simulink model "pid_adrc_duibi"  (R2023b)
settings: Solver=VariableStepAuto  StartTime=0.0  StopTime=10.0  RelTol=1e-3
values from neighbouring files (symbols this model uses):
  gama = 0.003    [startup.m]
  ke = 78.4    [startup.m]
  kf = 96.0    (= 96)    [startup.m]
  kii = 1061*R    (= 19755.82)    [startup.m]
  kiv = kpv*100    (= 7015.3125)    [startup.m]
  kp = 150    [startup.m]
  kpi = 1061*L    (= 16265.13)    [startup.m]
  kpv = 100*6*J/(kf)    (= 70.153125)    [startup.m]
  L = 15.33    [startup.m]
  R = 18.62    [startup.m]
  r = 10    [startup.m]
  tao = 0.003    [startup.m]
  U = m2^2*y^2+2*m1*m2*y^2+I1*(m1+m2)    [startup.m]
undefined symbols (not defined in the file or in its folder): sigbuilder_block
libraries: slpidlib x42, simulink x18
(part 1 of 2)
settings Model: Creator=CAE_B7  LastModifiedBy=Keaton
settings SolverCC: AlgebraicLoopSolver=TrustRegion
settings DataIOCC: ReturnWorkspaceOutputs=off
settings DebuggingCC: UnconnectedInputMsg=warning  UnconnectedOutputMsg=warning  UnconnectedLineMsg=warning  ArithmeticOperatorsInVariantConditions=warning
settings ModelReferenceCC: EnableRefExpFcnMdlSchedulingChecks=on
settings SFSimCC: SimUseLocalCustomCode=off  CustomCodeUndefinedFunction=UseInterfaceOnly
settings RTWCC: RTWUseLocalCustomCode=off

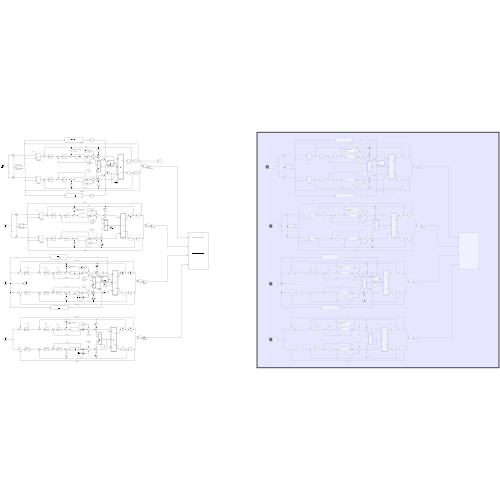
[thumbnail: Simulink's stored preview of the top-level diagram]
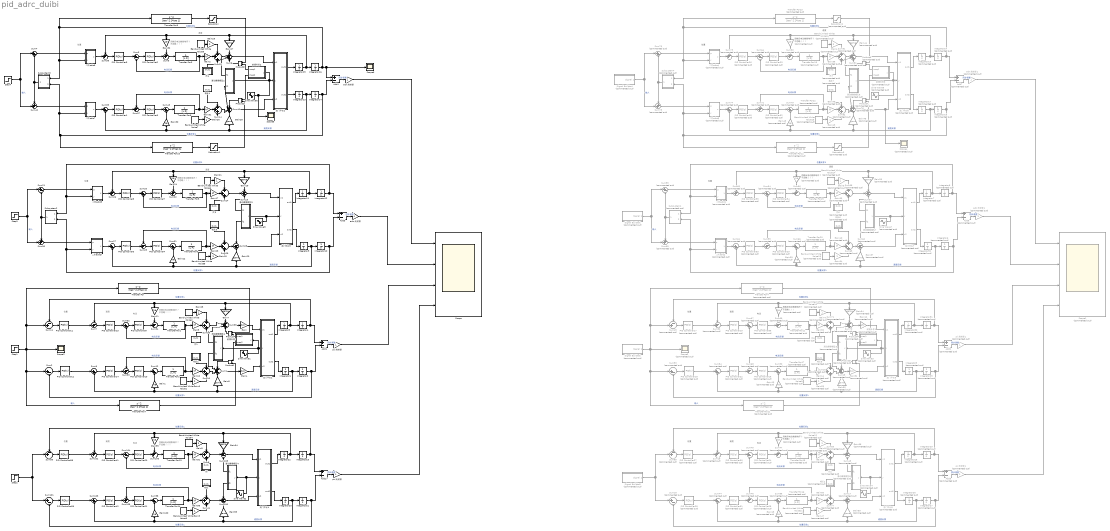
== system pid_adrc_duibi ==
  note: 速度
  note: 位置
  note: 忽略反电动势影响不？
      | 不忽略！！！
  note: 忽略反电动势影响不？
      | 不忽略！！！
  note: 忽略反电动势影响不？
      | 不忽略！！！
  note: 电流
  note: 速度
  note: 位置
  note: 位置
  note: 电流
  note: 速度
  note: 速度
  note: 位置
  note: 忽略反电动势影响不？
      | 不忽略！！！
  note: 忽略反电动势影响不？
      | 不忽略！！！
  note: 位置
  note: 电流
  note: 速度
  note: 位置
  note: 速度
  note: 电流
  note: 速度
  note: 忽略反电动势影响不？
      | 不忽略！！！
  note: 位置
  note: 速度
  note: 忽略反电动势影响不？
      | 不忽略！！！
  note: 位置
  note: 忽略反电动势影响不？
      | 不忽略！！！
  Add{1,3..4,17} (4 alike) : Sum  Inputs=+-
  Add{2,5..7} (4 alike) : Sum  Commented=on  Inputs=+-
  Band-Limited White Noise{1,3,5,7} (4 alike) : simulink/Sources/Band-Limited White Noise  Cov=[0.0001]  Ts=0.0001  seed=[23342]
  Band-Limited White Noise{10,12,14,16} (4 alike) : simulink/Sources/Band-Limited White Noise  Commented=on  Cov=[0.0001]  Ts=0.0001  seed=[23341]
  Band-Limited White Noise{9,11,13,15} (4 alike) : simulink/Sources/Band-Limited White Noise  Commented=on  Cov=[0.0001]  Ts=0.0001  seed=[23342]
  Band-Limited White Noise{2,4,6,8} (4 alike) : simulink/Sources/Band-Limited White Noise  Cov=[0.0001]  Ts=0.0001  seed=[23341]
  Gain : Gain  Gain=1/U
  Gain{1,11,22,24,30,32,99..100} (8 alike) : Gain  Gain=ke
  Gain{2,5,10,17,23,31,92,98} (8 alike) : Gain  Gain=kf
  Gain12 : Gain  Commented=on  Gain=1/U
  Gain{13,15..16,39,41,48,50,61} (8 alike) : Gain  Commented=on  Gain=ke
  Gain{14,33,36,40,49,52,57,60} (8 alike) : Gain  Commented=on  Gain=kf
  Gain{3,6,9,18,21,25..26,29} (8 alike) : Gain
  Gain{7..8,19..20,27..28,94..95} (8 alike) : Gain  Gain=gama
  Gain{34,38,42..43,46..47,53,56} (8 alike) : Gain  Commented=on
  Gain{35,37,44..45,54..55,58..59} (8 alike) : Gain  Commented=on  Gain=gama
  Gain4 : Gain  Gain=1/U
  Gain51 : Gain  Commented=on  Gain=1/U
  Integrator{1..4,9..16,20..23} (16 alike) : Integrator
  Integrator{5..8,17..19,24..32} (16 alike) : Integrator  Commented=on
  PID Controller{1,3,6,8,13..14,41..42} (8 alike) : slpidlib/PID Controller  Controller=PID  Form=Parallel  TimeDomain=Continuous-time  UseExternalTs=off  SampleTime=-1  IntegratorMethod=Forward Euler  FilterMethod=Forward Euler  ControllerParametersSource=internal  P=kpv  I=kiv  UseKiTs=off  D=0  N=100  UseFilter=on  TunerSelectOption=Transfer Function Based (PID Tuner App)  InitialConditionSource=internal  InitialConditionForIntegrator=0  InitialConditionForFilter=0  DifferentiatorICPrevScaledInput=0  ExternalReset=none  TrackingMode=off  Kt=1  LimitOutput=off  SatLimitsSource=internal  UpperSaturationLimit=inf  LowerSaturationLimit=-inf  LinearizeAsGain=on  AntiWindupMode=none  Kb=1  LimitIntegrator=off  UpperIntegratorSaturationLimit=inf  LowerIntegratorSaturationLimit=-inf  POutMin=[]  POutMax=[]  IOutMin=[]  IOutMax=[]  DOutMin=[]  DOutMax=[]  NOutMin=[]  NOutMax=[]  SumOutMin=[]  SumOutMax=[]  SaturationOutMin=[]  SaturationOutMax=[]  PParamMin=[]  PParamMax=[]  IParamMin=[]  IParamMax=[]  DParamMin=[]  DParamMax=[]  NParamMin=[]  NParamMax=[]  KbParamMin=[]  KbParamMax=[]  KtParamMin=[]  KtParamMax=[]  KbOutMin=[]  KbOutMax=[]  KtOutMin=[]  KtOutMax=[]  IntegratorOutMin=[]  IntegratorOutMax=[]  FilterOutMin=[]  FilterOutMax=[]  SumI1OutMin=[]  SumI1OutMax=[]  SumI2OutMin=[]  SumI2OutMax=[]  SumI3OutMin=[]  SumI3OutMax=[]  SumI4OutMin=[]  SumI4OutMax=[]  SumDOutMin=[]  SumDOutMax=[]  DifferentiatorOutMin=[]  DifferentiatorOutMax=[]  FilterDiffOutCoefMin=[]  FilterDiffOutCoefMax=[]  ReciprocalOutMin=[]  ReciprocalOutMax=[]  SumDenOutMin=[]  SumDenOutMax=[]  SumNumOutMin=[]  SumNumOutMax=[]  DivideOutMin=[]  DivideOutMax=[]  UdiffTsProdOutMin=[]  UdiffTsProdOutMax=[]  NTsProdOutMin=[]  NTsProdOutMax=[]  UintegralTsProdOutMin=[]  UintegralTsProdOutMax=[]  UngainTsProdOutMin=[]  UngainTsProdOutMax=[]  ClampingZeroOutDataTypeStr=Inherit: Inherit via back propagation  ClampingZeroOutMin=[]  ClampingZeroOutMax=[]  FilterDenConstantOutDataTypeStr=Inherit: Inherit via back propagation  FilterDenConstantOutMin=[]  FilterDenConstantOutMax=[]  PCopyOutDataTypeStr=Inherit: Inherit via back propagation  PCopyOutMin=[]  PCopyOutMax=[]  NCopyOutDataTypeStr=Inherit: Inherit via back propagation  NCopyOutMin=[]  NCopyOutMax=[]  IntegratorContinuousStateAttributes=''  IntegratorStateMustResolveToSignalObject=off  IntegratorRTWStateStorageClass=Auto  FilterContinuousStateAttributes=''  FilterStateMustResolveToSignalObject=off  FilterRTWStateStorageClass=Auto  ParallelPVariant=InternalParameters  IdealPVariant=Disabled  IVariant=InternalParameters  DVariant=InternalParameters  IntegratorVariant=Continuous  SatVariant=Disabled  AWVariant=Passthrough  PCopyVariant=Disabled  TRVariant=Disabled  FdbkBlocksVariant=Forward  IdealPFdbkVariant=Disabled  SatFdbkVariant=Disabled  DerivativeFilterVariant=ContFilter  NVariant=InternalParameters  NCopyVariant=Disabled  FilterICVariant=InternalICsFilter  IntegratorICVariant=InternalICs  ExternalResetVariant=Disabled  TRSumVariant=Passthrough  SumFdbkVariant=Disabled  SumVariant=Sum_PID  TsampFilterVariant=InternalTs  TsampNgainVariant=Passthrough  TsampIntegralVariant=Disabled_SignalSpec  ExternalSaturationOutDataTypeStr=Inherit: Same as second input
  PID Controller{2,4..5,7,9..10,20..21} (8 alike) : slpidlib/PID Controller  Controller=PID  Form=Parallel  TimeDomain=Continuous-time  UseExternalTs=off  SampleTime=-1  IntegratorMethod=Forward Euler  FilterMethod=Forward Euler  ControllerParametersSource=internal  P=kpi  I=kii  UseKiTs=off  D=0  N=100  UseFilter=on  TunerSelectOption=Transfer Function Based (PID Tuner App)  InitialConditionSource=internal  InitialConditionForIntegrator=0  InitialConditionForFilter=0  DifferentiatorICPrevScaledInput=0  ExternalReset=none  TrackingMode=off  Kt=1  LimitOutput=off  SatLimitsSource=internal  UpperSaturationLimit=inf  LowerSaturationLimit=-inf  LinearizeAsGain=on  AntiWindupMode=none  Kb=1  LimitIntegrator=off  UpperIntegratorSaturationLimit=inf  LowerIntegratorSaturationLimit=-inf  POutMin=[]  POutMax=[]  IOutMin=[]  IOutMax=[]  DOutMin=[]  DOutMax=[]  NOutMin=[]  NOutMax=[]  SumOutMin=[]  SumOutMax=[]  SaturationOutMin=[]  SaturationOutMax=[]  PParamMin=[]  PParamMax=[]  IParamMin=[]  IParamMax=[]  DParamMin=[]  DParamMax=[]  NParamMin=[]  NParamMax=[]  KbParamMin=[]  KbParamMax=[]  KtParamMin=[]  KtParamMax=[]  KbOutMin=[]  KbOutMax=[]  KtOutMin=[]  KtOutMax=[]  IntegratorOutMin=[]  IntegratorOutMax=[]  FilterOutMin=[]  FilterOutMax=[]  SumI1OutMin=[]  SumI1OutMax=[]  SumI2OutMin=[]  SumI2OutMax=[]  SumI3OutMin=[]  SumI3OutMax=[]  SumI4OutMin=[]  SumI4OutMax=[]  SumDOutMin=[]  SumDOutMax=[]  DifferentiatorOutMin=[]  DifferentiatorOutMax=[]  FilterDiffOutCoefMin=[]  FilterDiffOutCoefMax=[]  ReciprocalOutMin=[]  ReciprocalOutMax=[]  SumDenOutMin=[]  SumDenOutMax=[]  SumNumOutMin=[]  SumNumOutMax=[]  DivideOutMin=[]  DivideOutMax=[]  UdiffTsProdOutMin=[]  UdiffTsProdOutMax=[]  NTsProdOutMin=[]  NTsProdOutMax=[]  UintegralTsProdOutMin=[]  UintegralTsProdOutMax=[]  UngainTsProdOutMin=[]  UngainTsProdOutMax=[]  ClampingZeroOutDataTypeStr=Inherit: Inherit via back propagation  ClampingZeroOutMin=[]  ClampingZeroOutMax=[]  FilterDenConstantOutDataTypeStr=Inherit: Inherit via back propagation  FilterDenConstantOutMin=[]  FilterDenConstantOutMax=[]  PCopyOutDataTypeStr=Inherit: Inherit via back propagation  PCopyOutMin=[]  PCopyOutMax=[]  NCopyOutDataTypeStr=Inherit: Inherit via back propagation  NCopyOutMin=[]  NCopyOutMax=[]  IntegratorContinuousStateAttributes=''  IntegratorStateMustResolveToSignalObject=off  IntegratorRTWStateStorageClass=Auto  FilterContinuousStateAttributes=''  FilterStateMustResolveToSignalObject=off  FilterRTWStateStorageClass=Auto  ParallelPVariant=InternalParameters  IdealPVariant=Disabled  IVariant=InternalParameters  DVariant=InternalParameters  IntegratorVariant=Continuous  SatVariant=Disabled  AWVariant=Passthrough  PCopyVariant=Disabled  TRVariant=Disabled  FdbkBlocksVariant=Forward  IdealPFdbkVariant=Disabled  SatFdbkVariant=Disabled  DerivativeFilterVariant=ContFilter  NVariant=InternalParameters  NCopyVariant=Disabled  FilterICVariant=InternalICsFilter  IntegratorICVariant=InternalICs  ExternalResetVariant=Disabled  TRSumVariant=Passthrough  SumFdbkVariant=Disabled  SumVariant=Sum_PID  TsampFilterVariant=InternalTs  TsampNgainVariant=Passthrough  TsampIntegralVariant=Disabled_SignalSpec  ExternalSaturationOutDataTypeStr=Inherit: Same as second input
  PID Controller11 : slpidlib/PID Controller  Controller=PID  Form=Parallel  TimeDomain=Continuous-time  UseExternalTs=off  SampleTime=-1  IntegratorMethod=Forward Euler  FilterMethod=Forward Euler  ControllerParametersSource=internal  P=kp  I=0  UseKiTs=off  D=0  N=100  UseFilter=on  TunerSelectOption=Transfer Function Based (PID Tuner App)  InitialConditionSource=internal  InitialConditionForIntegrator=0  InitialConditionForFilter=0  DifferentiatorICPrevScaledInput=0  ExternalReset=none  TrackingMode=off  Kt=1  LimitOutput=off  SatLimitsSource=internal  UpperSaturationLimit=inf  LowerSaturationLimit=-inf  LinearizeAsGain=on  AntiWindupMode=none  Kb=1  LimitIntegrator=off  UpperIntegratorSaturationLimit=inf  LowerIntegratorSaturationLimit=-inf  POutMin=[]  POutMax=[]  IOutMin=[]  IOutMax=[]  DOutMin=[]  DOutMax=[]  NOutMin=[]  NOutMax=[]  SumOutMin=[]  SumOutMax=[]  SaturationOutMin=[]  SaturationOutMax=[]  PParamMin=[]  PParamMax=[]  IParamMin=[]  IParamMax=[]  DParamMin=[]  DParamMax=[]  NParamMin=[]  NParamMax=[]  KbParamMin=[]  KbParamMax=[]  KtParamMin=[]  KtParamMax=[]  KbOutMin=[]  KbOutMax=[]  KtOutMin=[]  KtOutMax=[]  IntegratorOutMin=[]  IntegratorOutMax=[]  FilterOutMin=[]  FilterOutMax=[]  SumI1OutMin=[]  SumI1OutMax=[]  SumI2OutMin=[]  SumI2OutMax=[]  SumI3OutMin=[]  SumI3OutMax=[]  SumI4OutMin=[]  SumI4OutMax=[]  SumDOutMin=[]  SumDOutMax=[]  DifferentiatorOutMin=[]  DifferentiatorOutMax=[]  FilterDiffOutCoefMin=[]  FilterDiffOutCoefMax=[]  ReciprocalOutMin=[]  ReciprocalOutMax=[]  SumDenOutMin=[]  SumDenOutMax=[]  SumNumOutMin=[]  SumNumOutMax=[]  DivideOutMin=[]  DivideOutMax=[]  UdiffTsProdOutMin=[]  UdiffTsProdOutMax=[]  NTsProdOutMin=[]  NTsProdOutMax=[]  UintegralTsProdOutMin=[]  UintegralTsProdOutMax=[]  UngainTsProdOutMin=[]  UngainTsProdOutMax=[]  ClampingZeroOutDataTypeStr=Inherit: Inherit via back propagation  ClampingZeroOutMin=[]  ClampingZeroOutMax=[]  FilterDenConstantOutDataTypeStr=Inherit: Inherit via back propagation  FilterDenConstantOutMin=[]  FilterDenConstantOutMax=[]  PCopyOutDataTypeStr=Inherit: Inherit via back propagation  PCopyOutMin=[]  PCopyOutMax=[]  NCopyOutDataTypeStr=Inherit: Inherit via back propagation  NCopyOutMin=[]  NCopyOutMax=[]  IntegratorContinuousStateAttributes=''  IntegratorStateMustResolveToSignalObject=off  IntegratorRTWStateStorageClass=Auto  FilterContinuousStateAttributes=''  FilterStateMustResolveToSignalObject=off  FilterRTWStateStorageClass=Auto  ParallelPVariant=InternalParameters  IdealPVariant=Disabled  IVariant=InternalParameters  DVariant=InternalParameters  IntegratorVariant=Continuous  SatVariant=Disabled  AWVariant=Passthrough  PCopyVariant=Disabled  TRVariant=Disabled  FdbkBlocksVariant=Forward  IdealPFdbkVariant=Disabled  SatFdbkVariant=Disabled  DerivativeFilterVariant=ContFilter  NVariant=InternalParameters  NCopyVariant=Disabled  FilterICVariant=InternalICsFilter  IntegratorICVariant=InternalICs  ExternalResetVariant=Disabled  TRSumVariant=Passthrough  SumFdbkVariant=Disabled  SumVariant=Sum_PID  TsampFilterVariant=InternalTs  TsampNgainVariant=Passthrough  TsampIntegralVariant=Disabled_SignalSpec  ExternalSaturationOutDataTypeStr=Inherit: Same as second input
  PID Controller12 : slpidlib/PID Controller  Controller=PID  Form=Parallel  TimeDomain=Continuous-time  UseExternalTs=off  SampleTime=-1  IntegratorMethod=Forward Euler  FilterMethod=Forward Euler  ControllerParametersSource=internal  P=kp  I=0  UseKiTs=off  D=0  N=95.162581964040484  UseFilter=on  TunerSelectOption=Transfer Function Based (PID Tuner App)  InitialConditionSource=internal  InitialConditionForIntegrator=0  InitialConditionForFilter=0  DifferentiatorICPrevScaledInput=0  ExternalReset=none  TrackingMode=off  Kt=1  LimitOutput=off  SatLimitsSource=internal  UpperSaturationLimit=inf  LowerSaturationLimit=-inf  LinearizeAsGain=on  AntiWindupMode=none  Kb=1  LimitIntegrator=off  UpperIntegratorSaturationLimit=inf  LowerIntegratorSaturationLimit=-inf  POutMin=[]  POutMax=[]  IOutMin=[]  IOutMax=[]  DOutMin=[]  DOutMax=[]  NOutMin=[]  NOutMax=[]  SumOutMin=[]  SumOutMax=[]  SaturationOutMin=[]  SaturationOutMax=[]  PParamMin=[]  PParamMax=[]  IParamMin=[]  IParamMax=[]  DParamMin=[]  DParamMax=[]  NParamMin=[]  NParamMax=[]  KbParamMin=[]  KbParamMax=[]  KtParamMin=[]  KtParamMax=[]  KbOutMin=[]  KbOutMax=[]  KtOutMin=[]  KtOutMax=[]  IntegratorOutMin=[]  IntegratorOutMax=[]  FilterOutMin=[]  FilterOutMax=[]  SumI1OutMin=[]  SumI1OutMax=[]  SumI2OutMin=[]  SumI2OutMax=[]  SumI3OutMin=[]  SumI3OutMax=[]  SumI4OutMin=[]  SumI4OutMax=[]  SumDOutMin=[]  SumDOutMax=[]  DifferentiatorOutMin=[]  DifferentiatorOutMax=[]  FilterDiffOutCoefMin=[]  FilterDiffOutCoefMax=[]  ReciprocalOutMin=[]  ReciprocalOutMax=[]  SumDenOutMin=[]  SumDenOutMax=[]  SumNumOutMin=[]  SumNumOutMax=[]  DivideOutMin=[]  DivideOutMax=[]  UdiffTsProdOutMin=[]  UdiffTsProdOutMax=[]  NTsProdOutMin=[]  NTsProdOutMax=[]  UintegralTsProdOutMin=[]  UintegralTsProdOutMax=[]  UngainTsProdOutMin=[]  UngainTsProdOutMax=[]  ClampingZeroOutDataTypeStr=Inherit: Inherit via back propagation  ClampingZeroOutMin=[]  ClampingZeroOutMax=[]  FilterDenConstantOutDataTypeStr=Inherit: Inherit via back propagation  FilterDenConstantOutMin=[]  FilterDenConstantOutMax=[]  PCopyOutDataTypeStr=Inherit: Inherit via back propagation  PCopyOutMin=[]  PCopyOutMax=[]  NCopyOutDataTypeStr=Inherit: Inherit via back propagation  NCopyOutMin=[]  NCopyOutMax=[]  IntegratorContinuousStateAttributes=''  IntegratorStateMustResolveToSignalObject=off  IntegratorRTWStateStorageClass=Auto  FilterContinuousStateAttributes=''  FilterStateMustResolveToSignalObject=off  FilterRTWStateStorageClass=Auto  ParallelPVariant=InternalParameters  IdealPVariant=Disabled  IVariant=InternalParameters  DVariant=InternalParameters  IntegratorVariant=Continuous  SatVariant=Disabled  AWVariant=Passthrough  PCopyVariant=Disabled  TRVariant=Disabled  FdbkBlocksVariant=Forward  IdealPFdbkVariant=Disabled  SatFdbkVariant=Disabled  DerivativeFilterVariant=ContFilter  NVariant=InternalParameters  NCopyVariant=Disabled  FilterICVariant=InternalICsFilter  IntegratorICVariant=InternalICs  ExternalResetVariant=Disabled  TRSumVariant=Passthrough  SumFdbkVariant=Disabled  SumVariant=Sum_PID  TsampFilterVariant=InternalTs  TsampNgainVariant=Passthrough  TsampIntegralVariant=Disabled_SignalSpec  ExternalSaturationOutDataTypeStr=Inherit: Same as second input
  PID Controller{15,19,22,26,30..31,33,35} (8 alike) : slpidlib/PID Controller  Commented=on  Controller=PID  Form=Parallel  TimeDomain=Continuous-time  UseExternalTs=off  SampleTime=-1  IntegratorMethod=Forward Euler  FilterMethod=Forward Euler  ControllerParametersSource=internal  P=kpv  I=kiv  UseKiTs=off  D=0  N=100  UseFilter=on  TunerSelectOption=Transfer Function Based (PID Tuner App)  InitialConditionSource=internal  InitialConditionForIntegrator=0  InitialConditionForFilter=0  DifferentiatorICPrevScaledInput=0  ExternalReset=none  TrackingMode=off  Kt=1  LimitOutput=off  SatLimitsSource=internal  UpperSaturationLimit=inf  LowerSaturationLimit=-inf  LinearizeAsGain=on  AntiWindupMode=none  Kb=1  LimitIntegrator=off  UpperIntegratorSaturationLimit=inf  LowerIntegratorSaturationLimit=-inf  POutMin=[]  POutMax=[]  IOutMin=[]  IOutMax=[]  DOutMin=[]  DOutMax=[]  NOutMin=[]  NOutMax=[]  SumOutMin=[]  SumOutMax=[]  SaturationOutMin=[]  SaturationOutMax=[]  PParamMin=[]  PParamMax=[]  IParamMin=[]  IParamMax=[]  DParamMin=[]  DParamMax=[]  NParamMin=[]  NParamMax=[]  KbParamMin=[]  KbParamMax=[]  KtParamMin=[]  KtParamMax=[]  KbOutMin=[]  KbOutMax=[]  KtOutMin=[]  KtOutMax=[]  IntegratorOutMin=[]  IntegratorOutMax=[]  FilterOutMin=[]  FilterOutMax=[]  SumI1OutMin=[]  SumI1OutMax=[]  SumI2OutMin=[]  SumI2OutMax=[]  SumI3OutMin=[]  SumI3OutMax=[]  SumI4OutMin=[]  SumI4OutMax=[]  SumDOutMin=[]  SumDOutMax=[]  DifferentiatorOutMin=[]  DifferentiatorOutMax=[]  FilterDiffOutCoefMin=[]  FilterDiffOutCoefMax=[]  ReciprocalOutMin=[]  ReciprocalOutMax=[]  SumDenOutMin=[]  SumDenOutMax=[]  SumNumOutMin=[]  SumNumOutMax=[]  DivideOutMin=[]  DivideOutMax=[]  UdiffTsProdOutMin=[]  UdiffTsProdOutMax=[]  NTsProdOutMin=[]  NTsProdOutMax=[]  UintegralTsProdOutMin=[]  UintegralTsProdOutMax=[]  UngainTsProdOutMin=[]  UngainTsProdOutMax=[]  ClampingZeroOutDataTypeStr=Inherit: Inherit via back propagation  ClampingZeroOutMin=[]  ClampingZeroOutMax=[]  FilterDenConstantOutDataTypeStr=Inherit: Inherit via back propagation  FilterDenConstantOutMin=[]  FilterDenConstantOutMax=[]  PCopyOutDataTypeStr=Inherit: Inherit via back propagation  PCopyOutMin=[]  PCopyOutMax=[]  NCopyOutDataTypeStr=Inherit: Inherit via back propagation  NCopyOutMin=[]  NCopyOutMax=[]  IntegratorContinuousStateAttributes=''  IntegratorStateMustResolveToSignalObject=off  IntegratorRTWStateStorageClass=Auto  FilterContinuousStateAttributes=''  FilterStateMustResolveToSignalObject=off  FilterRTWStateStorageClass=Auto  ParallelPVariant=InternalParameters  IdealPVariant=Disabled  IVariant=InternalParameters  DVariant=InternalParameters  IntegratorVariant=Continuous  SatVariant=Disabled  AWVariant=Passthrough  PCopyVariant=Disabled  TRVariant=Disabled  FdbkBlocksVariant=Forward  IdealPFdbkVariant=Disabled  SatFdbkVariant=Disabled  DerivativeFilterVariant=ContFilter  NVariant=InternalParameters  NCopyVariant=Disabled  FilterICVariant=InternalICsFilter  IntegratorICVariant=InternalICs  ExternalResetVariant=Disabled  TRSumVariant=Passthrough  SumFdbkVariant=Disabled  SumVariant=Sum_PID  TsampFilterVariant=InternalTs  TsampNgainVariant=Passthrough  TsampIntegralVariant=Disabled_SignalSpec  ExternalSaturationOutDataTypeStr=Inherit: Same as second input
  PID Controller{16,23..25,29,32,34,36} (8 alike) : slpidlib/PID Controller  Commented=on  Controller=PID  Form=Parallel  TimeDomain=Continuous-time  UseExternalTs=off  SampleTime=-1  IntegratorMethod=Forward Euler  FilterMethod=Forward Euler  ControllerParametersSource=internal  P=kpi  I=kii  UseKiTs=off  D=0  N=100  UseFilter=on  TunerSelectOption=Transfer Function Based (PID Tuner App)  InitialConditionSource=internal  InitialConditionForIntegrator=0  InitialConditionForFilter=0  DifferentiatorICPrevScaledInput=0  ExternalReset=none  TrackingMode=off  Kt=1  LimitOutput=off  SatLimitsSource=internal  UpperSaturationLimit=inf  LowerSaturationLimit=-inf  LinearizeAsGain=on  AntiWindupMode=none  Kb=1  LimitIntegrator=off  UpperIntegratorSaturationLimit=inf  LowerIntegratorSaturationLimit=-inf  POutMin=[]  POutMax=[]  IOutMin=[]  IOutMax=[]  DOutMin=[]  DOutMax=[]  NOutMin=[]  NOutMax=[]  SumOutMin=[]  SumOutMax=[]  SaturationOutMin=[]  SaturationOutMax=[]  PParamMin=[]  PParamMax=[]  IParamMin=[]  IParamMax=[]  DParamMin=[]  DParamMax=[]  NParamMin=[]  NParamMax=[]  KbParamMin=[]  KbParamMax=[]  KtParamMin=[]  KtParamMax=[]  KbOutMin=[]  KbOutMax=[]  KtOutMin=[]  KtOutMax=[]  IntegratorOutMin=[]  IntegratorOutMax=[]  FilterOutMin=[]  FilterOutMax=[]  SumI1OutMin=[]  SumI1OutMax=[]  SumI2OutMin=[]  SumI2OutMax=[]  SumI3OutMin=[]  SumI3OutMax=[]  SumI4OutMin=[]  SumI4OutMax=[]  SumDOutMin=[]  SumDOutMax=[]  DifferentiatorOutMin=[]  DifferentiatorOutMax=[]  FilterDiffOutCoefMin=[]  FilterDiffOutCoefMax=[]  ReciprocalOutMin=[]  ReciprocalOutMax=[]  SumDenOutMin=[]  SumDenOutMax=[]  SumNumOutMin=[]  SumNumOutMax=[]  DivideOutMin=[]  DivideOutMax=[]  UdiffTsProdOutMin=[]  UdiffTsProdOutMax=[]  NTsProdOutMin=[]  NTsProdOutMax=[]  UintegralTsProdOutMin=[]  UintegralTsProdOutMax=[]  UngainTsProdOutMin=[]  UngainTsProdOutMax=[]  ClampingZeroOutDataTypeStr=Inherit: Inherit via back propagation  ClampingZeroOutMin=[]  ClampingZeroOutMax=[]  FilterDenConstantOutDataTypeStr=Inherit: Inherit via back propagation  FilterDenConstantOutMin=[]  FilterDenConstantOutMax=[]  PCopyOutDataTypeStr=Inherit: Inherit via back propagation  PCopyOutMin=[]  PCopyOutMax=[]  NCopyOutDataTypeStr=Inherit: Inherit via back propagation  NCopyOutMin=[]  NCopyOutMax=[]  IntegratorContinuousStateAttributes=''  IntegratorStateMustResolveToSignalObject=off  IntegratorRTWStateStorageClass=Auto  FilterContinuousStateAttributes=''  FilterStateMustResolveToSignalObject=off  FilterRTWStateStorageClass=Auto  ParallelPVariant=InternalParameters  IdealPVariant=Disabled  IVariant=InternalParameters  DVariant=InternalParameters  IntegratorVariant=Continuous  SatVariant=Disabled  AWVariant=Passthrough  PCopyVariant=Disabled  TRVariant=Disabled  FdbkBlocksVariant=Forward  IdealPFdbkVariant=Disabled  SatFdbkVariant=Disabled  DerivativeFilterVariant=ContFilter  NVariant=InternalParameters  NCopyVariant=Disabled  FilterICVariant=InternalICsFilter  IntegratorICVariant=InternalICs  ExternalResetVariant=Disabled  TRSumVariant=Passthrough  SumFdbkVariant=Disabled  SumVariant=Sum_PID  TsampFilterVariant=InternalTs  TsampNgainVariant=Passthrough  TsampIntegralVariant=Disabled_SignalSpec  ExternalSaturationOutDataTypeStr=Inherit: Same as second input
  PID Controller17 : slpidlib/PID Controller  Commented=on  Controller=PID  Form=Parallel  TimeDomain=Continuous-time  UseExternalTs=off  SampleTime=-1  IntegratorMethod=Forward Euler  FilterMethod=Forward Euler  ControllerParametersSource=internal  P=kp  I=0  UseKiTs=off  D=0  N=100  UseFilter=on  TunerSelectOption=Transfer Function Based (PID Tuner App)  InitialConditionSource=internal  InitialConditionForIntegrator=0  InitialConditionForFilter=0  DifferentiatorICPrevScaledInput=0  ExternalReset=none  TrackingMode=off  Kt=1  LimitOutput=off  SatLimitsSource=internal  UpperSaturationLimit=inf  LowerSaturationLimit=-inf  LinearizeAsGain=on  AntiWindupMode=none  Kb=1  LimitIntegrator=off  UpperIntegratorSaturationLimit=inf  LowerIntegratorSaturationLimit=-inf  POutMin=[]  POutMax=[]  IOutMin=[]  IOutMax=[]  DOutMin=[]  DOutMax=[]  NOutMin=[]  NOutMax=[]  SumOutMin=[]  SumOutMax=[]  SaturationOutMin=[]  SaturationOutMax=[]  PParamMin=[]  PParamMax=[]  IParamMin=[]  IParamMax=[]  DParamMin=[]  DParamMax=[]  NParamMin=[]  NParamMax=[]  KbParamMin=[]  KbParamMax=[]  KtParamMin=[]  KtParamMax=[]  KbOutMin=[]  KbOutMax=[]  KtOutMin=[]  KtOutMax=[]  IntegratorOutMin=[]  IntegratorOutMax=[]  FilterOutMin=[]  FilterOutMax=[]  SumI1OutMin=[]  SumI1OutMax=[]  SumI2OutMin=[]  SumI2OutMax=[]  SumI3OutMin=[]  SumI3OutMax=[]  SumI4OutMin=[]  SumI4OutMax=[]  SumDOutMin=[]  SumDOutMax=[]  DifferentiatorOutMin=[]  DifferentiatorOutMax=[]  FilterDiffOutCoefMin=[]  FilterDiffOutCoefMax=[]  ReciprocalOutMin=[]  ReciprocalOutMax=[]  SumDenOutMin=[]  SumDenOutMax=[]  SumNumOutMin=[]  SumNumOutMax=[]  DivideOutMin=[]  DivideOutMax=[]  UdiffTsProdOutMin=[]  UdiffTsProdOutMax=[]  NTsProdOutMin=[]  NTsProdOutMax=[]  UintegralTsProdOutMin=[]  UintegralTsProdOutMax=[]  UngainTsProdOutMin=[]  UngainTsProdOutMax=[]  ClampingZeroOutDataTypeStr=Inherit: Inherit via back propagation  ClampingZeroOutMin=[]  ClampingZeroOutMax=[]  FilterDenConstantOutDataTypeStr=Inherit: Inherit via back propagation  FilterDenConstantOutMin=[]  FilterDenConstantOutMax=[]  PCopyOutDataTypeStr=Inherit: Inherit via back propagation  PCopyOutMin=[]  PCopyOutMax=[]  NCopyOutDataTypeStr=Inherit: Inherit via back propagation  NCopyOutMin=[]  NCopyOutMax=[]  IntegratorContinuousStateAttributes=''  IntegratorStateMustResolveToSignalObject=off  IntegratorRTWStateStorageClass=Auto  FilterContinuousStateAttributes=''  FilterStateMustResolveToSignalObject=off  FilterRTWStateStorageClass=Auto  ParallelPVariant=InternalParameters  IdealPVariant=Disabled  IVariant=InternalParameters  DVariant=InternalParameters  IntegratorVariant=Continuous  SatVariant=Disabled  AWVariant=Passthrough  PCopyVariant=Disabled  TRVariant=Disabled  FdbkBlocksVariant=Forward  IdealPFdbkVariant=Disabled  SatFdbkVariant=Disabled  DerivativeFilterVariant=ContFilter  NVariant=InternalParameters  NCopyVariant=Disabled  FilterICVariant=InternalICsFilter  IntegratorICVariant=InternalICs  ExternalResetVariant=Disabled  TRSumVariant=Passthrough  SumFdbkVariant=Disabled  SumVariant=Sum_PID  TsampFilterVariant=InternalTs  TsampNgainVariant=Passthrough  TsampIntegralVariant=Disabled_SignalSpec  ExternalSaturationOutDataTypeStr=Inherit: Same as second input
  PID Controller18 : slpidlib/PID Controller  Commented=on  Controller=PID  Form=Parallel  TimeDomain=Continuous-time  UseExternalTs=off  SampleTime=-1  IntegratorMethod=Forward Euler  FilterMethod=Forward Euler  ControllerParametersSource=internal  P=kp  I=0  UseKiTs=off  D=0  N=95.162581964040484  UseFilter=on  TunerSelectOption=Transfer Function Based (PID Tuner App)  InitialConditionSource=internal  InitialConditionForIntegrator=0  InitialConditionForFilter=0  DifferentiatorICPrevScaledInput=0  ExternalReset=none  TrackingMode=off  Kt=1  LimitOutput=off  SatLimitsSource=internal  UpperSaturationLimit=inf  LowerSaturationLimit=-inf  LinearizeAsGain=on  AntiWindupMode=none  Kb=1  LimitIntegrator=off  UpperIntegratorSaturationLimit=inf  LowerIntegratorSaturationLimit=-inf  POutMin=[]  POutMax=[]  IOutMin=[]  IOutMax=[]  DOutMin=[]  DOutMax=[]  NOutMin=[]  NOutMax=[]  SumOutMin=[]  SumOutMax=[]  SaturationOutMin=[]  SaturationOutMax=[]  PParamMin=[]  PParamMax=[]  IParamMin=[]  IParamMax=[]  DParamMin=[]  DParamMax=[]  NParamMin=[]  NParamMax=[]  KbParamMin=[]  KbParamMax=[]  KtParamMin=[]  KtParamMax=[]  KbOutMin=[]  KbOutMax=[]  KtOutMin=[]  KtOutMax=[]  IntegratorOutMin=[]  IntegratorOutMax=[]  FilterOutMin=[]  FilterOutMax=[]  SumI1OutMin=[]  SumI1OutMax=[]  SumI2OutMin=[]  SumI2OutMax=[]  SumI3OutMin=[]  SumI3OutMax=[]  SumI4OutMin=[]  SumI4OutMax=[]  SumDOutMin=[]  SumDOutMax=[]  DifferentiatorOutMin=[]  DifferentiatorOutMax=[]  FilterDiffOutCoefMin=[]  FilterDiffOutCoefMax=[]  ReciprocalOutMin=[]  ReciprocalOutMax=[]  SumDenOutMin=[]  SumDenOutMax=[]  SumNumOutMin=[]  SumNumOutMax=[]  DivideOutMin=[]  DivideOutMax=[]  UdiffTsProdOutMin=[]  UdiffTsProdOutMax=[]  NTsProdOutMin=[]  NTsProdOutMax=[]  UintegralTsProdOutMin=[]  UintegralTsProdOutMax=[]  UngainTsProdOutMin=[]  UngainTsProdOutMax=[]  ClampingZeroOutDataTypeStr=Inherit: Inherit via back propagation  ClampingZeroOutMin=[]  ClampingZeroOutMax=[]  FilterDenConstantOutDataTypeStr=Inherit: Inherit via back propagation  FilterDenConstantOutMin=[]  FilterDenConstantOutMax=[]  PCopyOutDataTypeStr=Inherit: Inherit via back propagation  PCopyOutMin=[]  PCopyOutMax=[]  NCopyOutDataTypeStr=Inherit: Inherit via back propagation  NCopyOutMin=[]  NCopyOutMax=[]  IntegratorContinuousStateAttributes=''  IntegratorStateMustResolveToSignalObject=off  IntegratorRTWStateStorageClass=Auto  FilterContinuousStateAttributes=''  FilterStateMustResolveToSignalObject=off  FilterRTWStateStorageClass=Auto  ParallelPVariant=InternalParameters  IdealPVariant=Disabled  IVariant=InternalParameters  DVariant=InternalParameters  IntegratorVariant=Continuous  SatVariant=Disabled  AWVariant=Passthrough  PCopyVariant=Disabled  TRVariant=Disabled  FdbkBlocksVariant=Forward  IdealPFdbkVariant=Disabled  SatFdbkVariant=Disabled  DerivativeFilterVariant=ContFilter  NVariant=InternalParameters  NCopyVariant=Disabled  FilterICVariant=InternalICsFilter  IntegratorICVariant=InternalICs  ExternalResetVariant=Disabled  TRSumVariant=Passthrough  SumFdbkVariant=Disabled  SumVariant=Sum_PID  TsampFilterVariant=InternalTs  TsampNgainVariant=Passthrough  TsampIntegralVariant=Disabled_SignalSpec  ExternalSaturationOutDataTypeStr=Inherit: Same as second input
  PID Controller27 : slpidlib/PID Controller  Commented=on  Controller=PID  Form=Parallel  TimeDomain=Continuous-time  UseExternalTs=off  SampleTime=-1  IntegratorMethod=Forward Euler  FilterMethod=Forward Euler  ControllerParametersSource=internal  P=kp  I=0  UseKiTs=off  D=0  N=100  UseFilter=on  TunerSelectOption=Transfer Function Based (PID Tuner App)  InitialConditionSource=internal  InitialConditionForIntegrator=0  InitialConditionForFilter=0  DifferentiatorICPrevScaledInput=0  ExternalReset=none  TrackingMode=off  Kt=1  LimitOutput=off  SatLimitsSource=internal  UpperSaturationLimit=inf  LowerSaturationLimit=-inf  LinearizeAsGain=on  AntiWindupMode=none  Kb=1  LimitIntegrator=off  UpperIntegratorSaturationLimit=inf  LowerIntegratorSaturationLimit=-inf  POutMin=[]  POutMax=[]  IOutMin=[]  IOutMax=[]  DOutMin=[]  DOutMax=[]  NOutMin=[]  NOutMax=[]  SumOutMin=[]  SumOutMax=[]  SaturationOutMin=[]  SaturationOutMax=[]  PParamMin=[]  PParamMax=[]  IParamMin=[]  IParamMax=[]  DParamMin=[]  DParamMax=[]  NParamMin=[]  NParamMax=[]  KbParamMin=[]  KbParamMax=[]  KtParamMin=[]  KtParamMax=[]  KbOutMin=[]  KbOutMax=[]  KtOutMin=[]  KtOutMax=[]  IntegratorOutMin=[]  IntegratorOutMax=[]  FilterOutMin=[]  FilterOutMax=[]  SumI1OutMin=[]  SumI1OutMax=[]  SumI2OutMin=[]  SumI2OutMax=[]  SumI3OutMin=[]  SumI3OutMax=[]  SumI4OutMin=[]  SumI4OutMax=[]  SumDOutMin=[]  SumDOutMax=[]  DifferentiatorOutMin=[]  DifferentiatorOutMax=[]  FilterDiffOutCoefMin=[]  FilterDiffOutCoefMax=[]  ReciprocalOutMin=[]  ReciprocalOutMax=[]  SumDenOutMin=[]  SumDenOutMax=[]  SumNumOutMin=[]  SumNumOutMax=[]  DivideOutMin=[]  DivideOutMax=[]  UdiffTsProdOutMin=[]  UdiffTsProdOutMax=[]  NTsProdOutMin=[]  NTsProdOutMax=[]  UintegralTsProdOutMin=[]  UintegralTsProdOutMax=[]  UngainTsProdOutMin=[]  UngainTsProdOutMax=[]  ClampingZeroOutDataTypeStr=Inherit: Inherit via back propagation  ClampingZeroOutMin=[]  ClampingZeroOutMax=[]  FilterDenConstantOutDataTypeStr=Inherit: Inherit via back propagation  FilterDenConstantOutMin=[]  FilterDenConstantOutMax=[]  PCopyOutDataTypeStr=Inherit: Inherit via back propagation  PCopyOutMin=[]  PCopyOutMax=[]  NCopyOutDataTypeStr=Inherit: Inherit via back propagation  NCopyOutMin=[]  NCopyOutMax=[]  IntegratorContinuousStateAttributes=''  IntegratorStateMustResolveToSignalObject=off  IntegratorRTWStateStorageClass=Auto  FilterContinuousStateAttributes=''  FilterStateMustResolveToSignalObject=off  FilterRTWStateStorageClass=Auto  ParallelPVariant=InternalParameters  IdealPVariant=Disabled  IVariant=InternalParameters  DVariant=InternalParameters  IntegratorVariant=Continuous  SatVariant=Disabled  AWVariant=Passthrough  PCopyVariant=Disabled  TRVariant=Disabled  FdbkBlocksVariant=Forward  IdealPFdbkVariant=Disabled  SatFdbkVariant=Disabled  DerivativeFilterVariant=ContFilter  NVariant=InternalParameters  NCopyVariant=Disabled  FilterICVariant=InternalICsFilter  IntegratorICVariant=InternalICs  ExternalResetVariant=Disabled  TRSumVariant=Passthrough  SumFdbkVariant=Disabled  SumVariant=Sum_PID  TsampFilterVariant=InternalTs  TsampNgainVariant=Passthrough  TsampIntegralVariant=Disabled_SignalSpec  ExternalSaturationOutDataTypeStr=Inherit: Same as second input
  PID Controller28 : slpidlib/PID Controller  Commented=on  Controller=PID  Form=Parallel  TimeDomain=Continuous-time  UseExternalTs=off  SampleTime=-1  IntegratorMethod=Forward Euler  FilterMethod=Forward Euler  ControllerParametersSource=internal  P=kp  I=0  UseKiTs=off  D=0  N=95.162581964040484  UseFilter=on  TunerSelectOption=Transfer Function Based (PID Tuner App)  InitialConditionSource=internal  InitialConditionForIntegrator=0  InitialConditionForFilter=0  DifferentiatorICPrevScaledInput=0  ExternalReset=none  TrackingMode=off  Kt=1  LimitOutput=off  SatLimitsSource=internal  UpperSaturationLimit=inf  LowerSaturationLimit=-inf  LinearizeAsGain=on  AntiWindupMode=none  Kb=1  LimitIntegrator=off  UpperIntegratorSaturationLimit=inf  LowerIntegratorSaturationLimit=-inf  POutMin=[]  POutMax=[]  IOutMin=[]  IOutMax=[]  DOutMin=[]  DOutMax=[]  NOutMin=[]  NOutMax=[]  SumOutMin=[]  SumOutMax=[]  SaturationOutMin=[]  SaturationOutMax=[]  PParamMin=[]  PParamMax=[]  IParamMin=[]  IParamMax=[]  DParamMin=[]  DParamMax=[]  NParamMin=[]  NParamMax=[]  KbParamMin=[]  KbParamMax=[]  KtParamMin=[]  KtParamMax=[]  KbOutMin=[]  KbOutMax=[]  KtOutMin=[]  KtOutMax=[]  IntegratorOutMin=[]  IntegratorOutMax=[]  FilterOutMin=[]  FilterOutMax=[]  SumI1OutMin=[]  SumI1OutMax=[]  SumI2OutMin=[]  SumI2OutMax=[]  SumI3OutMin=[]  SumI3OutMax=[]  SumI4OutMin=[]  SumI4OutMax=[]  SumDOutMin=[]  SumDOutMax=[]  DifferentiatorOutMin=[]  DifferentiatorOutMax=[]  FilterDiffOutCoefMin=[]  FilterDiffOutCoefMax=[]  ReciprocalOutMin=[]  ReciprocalOutMax=[]  SumDenOutMin=[]  SumDenOutMax=[]  SumNumOutMin=[]  SumNumOutMax=[]  DivideOutMin=[]  DivideOutMax=[]  UdiffTsProdOutMin=[]  UdiffTsProdOutMax=[]  NTsProdOutMin=[]  NTsProdOutMax=[]  UintegralTsProdOutMin=[]  UintegralTsProdOutMax=[]  UngainTsProdOutMin=[]  UngainTsProdOutMax=[]  ClampingZeroOutDataTypeStr=Inherit: Inherit via back propagation  ClampingZeroOutMin=[]  ClampingZeroOutMax=[]  FilterDenConstantOutDataTypeStr=Inherit: Inherit via back propagation  FilterDenConstantOutMin=[]  FilterDenConstantOutMax=[]  PCopyOutDataTypeStr=Inherit: Inherit via back propagation  PCopyOutMin=[]  PCopyOutMax=[]  NCopyOutDataTypeStr=Inherit: Inherit via back propagation  NCopyOutMin=[]  NCopyOutMax=[]  IntegratorContinuousStateAttributes=''  IntegratorStateMustResolveToSignalObject=off  IntegratorRTWStateStorageClass=Auto  FilterContinuousStateAttributes=''  FilterStateMustResolveToSignalObject=off  FilterRTWStateStorageClass=Auto  ParallelPVariant=InternalParameters  IdealPVariant=Disabled  IVariant=InternalParameters  DVariant=InternalParameters  IntegratorVariant=Continuous  SatVariant=Disabled  AWVariant=Passthrough  PCopyVariant=Disabled  TRVariant=Disabled  FdbkBlocksVariant=Forward  IdealPFdbkVariant=Disabled  SatFdbkVariant=Disabled  DerivativeFilterVariant=ContFilter  NVariant=InternalParameters  NCopyVariant=Disabled  FilterICVariant=InternalICsFilter  IntegratorICVariant=InternalICs  ExternalResetVariant=Disabled  TRSumVariant=Passthrough  SumFdbkVariant=Disabled  SumVariant=Sum_PID  TsampFilterVariant=InternalTs  TsampNgainVariant=Passthrough  TsampIntegralVariant=Disabled_SignalSpec  ExternalSaturationOutDataTypeStr=Inherit: Same as second input
  PID Controller38 : slpidlib/PID Controller  Controller=PID  Form=Parallel  TimeDomain=Continuous-time  UseExternalTs=off  SampleTime=-1  IntegratorMethod=Forward Euler  FilterMethod=Forward Euler  ControllerParametersSource=internal  P=kp  I=0  UseKiTs=off  D=0  N=100  UseFilter=on  TunerSelectOption=Transfer Function Based (PID Tuner App)  InitialConditionSource=internal  InitialConditionForIntegrator=0  InitialConditionForFilter=0  DifferentiatorICPrevScaledInput=0  ExternalReset=none  TrackingMode=off  Kt=1  LimitOutput=off  SatLimitsSource=internal  UpperSaturationLimit=inf  LowerSaturationLimit=-inf  LinearizeAsGain=on  AntiWindupMode=none  Kb=1  LimitIntegrator=off  UpperIntegratorSaturationLimit=inf  LowerIntegratorSaturationLimit=-inf  POutMin=[]  POutMax=[]  IOutMin=[]  IOutMax=[]  DOutMin=[]  DOutMax=[]  NOutMin=[]  NOutMax=[]  SumOutMin=[]  SumOutMax=[]  SaturationOutMin=[]  SaturationOutMax=[]  PParamMin=[]  PParamMax=[]  IParamMin=[]  IParamMax=[]  DParamMin=[]  DParamMax=[]  NParamMin=[]  NParamMax=[]  KbParamMin=[]  KbParamMax=[]  KtParamMin=[]  KtParamMax=[]  KbOutMin=[]  KbOutMax=[]  KtOutMin=[]  KtOutMax=[]  IntegratorOutMin=[]  IntegratorOutMax=[]  FilterOutMin=[]  FilterOutMax=[]  SumI1OutMin=[]  SumI1OutMax=[]  SumI2OutMin=[]  SumI2OutMax=[]  SumI3OutMin=[]  SumI3OutMax=[]  SumI4OutMin=[]  SumI4OutMax=[]  SumDOutMin=[]  SumDOutMax=[]  DifferentiatorOutMin=[]  DifferentiatorOutMax=[]  FilterDiffOutCoefMin=[]  FilterDiffOutCoefMax=[]  ReciprocalOutMin=[]  ReciprocalOutMax=[]  SumDenOutMin=[]  SumDenOutMax=[]  SumNumOutMin=[]  SumNumOutMax=[]  DivideOutMin=[]  DivideOutMax=[]  UdiffTsProdOutMin=[]  UdiffTsProdOutMax=[]  NTsProdOutMin=[]  NTsProdOutMax=[]  UintegralTsProdOutMin=[]  UintegralTsProdOutMax=[]  UngainTsProdOutMin=[]  UngainTsProdOutMax=[]  ClampingZeroOutDataTypeStr=Inherit: Inherit via back propagation  ClampingZeroOutMin=[]  ClampingZeroOutMax=[]  FilterDenConstantOutDataTypeStr=Inherit: Inherit via back propagation  FilterDenConstantOutMin=[]  FilterDenConstantOutMax=[]  PCopyOutDataTypeStr=Inherit: Inherit via back propagation  PCopyOutMin=[]  PCopyOutMax=[]  NCopyOutDataTypeStr=Inherit: Inherit via back propagation  NCopyOutMin=[]  NCopyOutMax=[]  IntegratorContinuousStateAttributes=''  IntegratorStateMustResolveToSignalObject=off  IntegratorRTWStateStorageClass=Auto  FilterContinuousStateAttributes=''  FilterStateMustResolveToSignalObject=off  FilterRTWStateStorageClass=Auto  ParallelPVariant=InternalParameters  IdealPVariant=Disabled  IVariant=InternalParameters  DVariant=InternalParameters  IntegratorVariant=Continuous  SatVariant=Disabled  AWVariant=Passthrough  PCopyVariant=Disabled  TRVariant=Disabled  FdbkBlocksVariant=Forward  IdealPFdbkVariant=Disabled  SatFdbkVariant=Disabled  DerivativeFilterVariant=ContFilter  NVariant=InternalParameters  NCopyVariant=Disabled  FilterICVariant=InternalICsFilter  IntegratorICVariant=InternalICs  ExternalResetVariant=Disabled  TRSumVariant=Passthrough  SumFdbkVariant=Disabled  SumVariant=Sum_PID  TsampFilterVariant=InternalTs  TsampNgainVariant=Passthrough  TsampIntegralVariant=Disabled_SignalSpec  ExternalSaturationOutDataTypeStr=Inherit: Same as second input
  PID Controller39 : slpidlib/PID Controller  Controller=PID  Form=Parallel  TimeDomain=Continuous-time  UseExternalTs=off  SampleTime=-1  IntegratorMethod=Forward Euler  FilterMethod=Forward Euler  ControllerParametersSource=internal  P=kp  I=0  UseKiTs=off  D=0  N=95.162581964040484  UseFilter=on  TunerSelectOption=Transfer Function Based (PID Tuner App)  InitialConditionSource=internal  InitialConditionForIntegrator=0  InitialConditionForFilter=0  DifferentiatorICPrevScaledInput=0  ExternalReset=none  TrackingMode=off  Kt=1  LimitOutput=off  SatLimitsSource=internal  UpperSaturationLimit=inf  LowerSaturationLimit=-inf  LinearizeAsGain=on  AntiWindupMode=none  Kb=1  LimitIntegrator=off  UpperIntegratorSaturationLimit=inf  LowerIntegratorSaturationLimit=-inf  POutMin=[]  POutMax=[]  IOutMin=[]  IOutMax=[]  DOutMin=[]  DOutMax=[]  NOutMin=[]  NOutMax=[]  SumOutMin=[]  SumOutMax=[]  SaturationOutMin=[]  SaturationOutMax=[]  PParamMin=[]  PParamMax=[]  IParamMin=[]  IParamMax=[]  DParamMin=[]  DParamMax=[]  NParamMin=[]  NParamMax=[]  KbParamMin=[]  KbParamMax=[]  KtParamMin=[]  KtParamMax=[]  KbOutMin=[]  KbOutMax=[]  KtOutMin=[]  KtOutMax=[]  IntegratorOutMin=[]  IntegratorOutMax=[]  FilterOutMin=[]  FilterOutMax=[]  SumI1OutMin=[]  SumI1OutMax=[]  SumI2OutMin=[]  SumI2OutMax=[]  SumI3OutMin=[]  SumI3OutMax=[]  SumI4OutMin=[]  SumI4OutMax=[]  SumDOutMin=[]  SumDOutMax=[]  DifferentiatorOutMin=[]  DifferentiatorOutMax=[]  FilterDiffOutCoefMin=[]  FilterDiffOutCoefMax=[]  ReciprocalOutMin=[]  ReciprocalOutMax=[]  SumDenOutMin=[]  SumDenOutMax=[]  SumNumOutMin=[]  SumNumOutMax=[]  DivideOutMin=[]  DivideOutMax=[]  UdiffTsProdOutMin=[]  UdiffTsProdOutMax=[]  NTsProdOutMin=[]  NTsProdOutMax=[]  UintegralTsProdOutMin=[]  UintegralTsProdOutMax=[]  UngainTsProdOutMin=[]  UngainTsProdOutMax=[]  ClampingZeroOutDataTypeStr=Inherit: Inherit via back propagation  ClampingZeroOutMin=[]  ClampingZeroOutMax=[]  FilterDenConstantOutDataTypeStr=Inherit: Inherit via back propagation  FilterDenConstantOutMin=[]  FilterDenConstantOutMax=[]  PCopyOutDataTypeStr=Inherit: Inherit via back propagation  PCopyOutMin=[]  PCopyOutMax=[]  NCopyOutDataTypeStr=Inherit: Inherit via back propagation  NCopyOutMin=[]  NCopyOutMax=[]  IntegratorContinuousStateAttributes=''  IntegratorStateMustResolveToSignalObject=off  IntegratorRTWStateStorageClass=Auto  FilterContinuousStateAttributes=''  FilterStateMustResolveToSignalObject=off  FilterRTWStateStorageClass=Auto  ParallelPVariant=InternalParameters  IdealPVariant=Disabled  IVariant=InternalParameters  DVariant=InternalParameters  IntegratorVariant=Continuous  SatVariant=Disabled  AWVariant=Passthrough  PCopyVariant=Disabled  TRVariant=Disabled  FdbkBlocksVariant=Forward  IdealPFdbkVariant=Disabled  SatFdbkVariant=Disabled  DerivativeFilterVariant=ContFilter  NVariant=InternalParameters  NCopyVariant=Disabled  FilterICVariant=InternalICsFilter  IntegratorICVariant=InternalICs  ExternalResetVariant=Disabled  TRSumVariant=Passthrough  SumFdbkVariant=Disabled  SumVariant=Sum_PID  TsampFilterVariant=InternalTs  TsampNgainVariant=Passthrough  TsampIntegralVariant=Disabled_SignalSpec  ExternalSaturationOutDataTypeStr=Inherit: Same as second input
  Product{,1..3} (4 alike) : Product
  Product{4..7} (4 alike) : Product  Commented=on
  Saturation : Saturate  UpperLimit=50  LowerLimit=-50
  Saturation1 : Saturate  UpperLimit=50  LowerLimit=-50
  Saturation2 : Saturate  Commented=on  UpperLimit=50  LowerLimit=-50
  Saturation3 : Saturate  Commented=on  UpperLimit=50  LowerLimit=-50
  Scope : Scope  NumInputPorts=4
  Scope1 : Scope  Commented=on  NumInputPorts=4
  Scope2 : Scope
  Scope3 : Scope  Commented=on
  Scope4 : Scope  Commented=on
  Scope5 : Scope
  Scope6 : Scope
  Signal Builder1 : Subsystem  Tag=STV Subsys  Commented=on  LoadFcn=sigbuilder_block('load');  StartFcn=sigbuilder_block('start');  StopFcn=sigbuilder_block('stop');  ClipboardFcn=sigbuilder_block('clipboard');  mask(Sigbuilder block){tuvar=[0:10]}
      mask help: Simulink:masks:SigbuilderBlock_MD
      mask init:
      | if ~strcmp(get_param(bdroot(gcbh),'SimulationStatus'),'stopped') tuvar = sigbuilder_block('maskInit'); end
      settings: CopyFcn=sigbuilder_block('copy');  DeleteFcn=sigbuilder_block('delete');  ModelCloseFcn=sigbuilder_block('modelClose');  PreSaveFcn=sigbuilder_block('preSave');  PauseFcn=sigbuilder_block('pause');  ContinueFcn=sigbuilder_block('continue');  NameChangeFcn=sigbuilder_block('namechange');  OpenFcn=sigbuilder_block('open',[437.6 199.2 550.4 400 ]);  CloseFcn=sigbuilder_block('close');
      mask Display: plot(0, 0, 100, 100,[2, 2, 32, 32, 2], [68, 8, 8, 68, 68],[32, 2], [38, 38], [32, 19, 2],[53, 60, 44], [32, 17, 17, 2],[16, 16, 31, 31]);txt = getActiveGroup(gcbh);text(2, 100, txt,'verticalAlignment', 'top');
  Signal Builder2 : Subsystem  Tag=STV Subsys  Commented=on  LoadFcn=sigbuilder_block('load');  StartFcn=sigbuilder_block('start');  StopFcn=sigbuilder_block('stop');  ClipboardFcn=sigbuilder_block('clipboard');  mask(Sigbuilder block){tuvar=[0:10]}
      mask help: Simulink:masks:SigbuilderBlock_MD
      mask init:
      | if ~strcmp(get_param(bdroot(gcbh),'SimulationStatus'),'stopped') tuvar = sigbuilder_block('maskInit'); end
      settings: CopyFcn=sigbuilder_block('copy');  DeleteFcn=sigbuilder_block('delete');  ModelCloseFcn=sigbuilder_block('modelClose');  PreSaveFcn=sigbuilder_block('preSave');  PauseFcn=sigbuilder_block('pause');  ContinueFcn=sigbuilder_block('continue');  NameChangeFcn=sigbuilder_block('namechange');  OpenFcn=sigbuilder_block('open',[437.6 199.2 550.4 400 ]);  CloseFcn=sigbuilder_block('close');
      mask Display: plot(0, 0, 100, 100,[2, 2, 32, 32, 2], [68, 8, 8, 68, 68],[32, 2], [38, 38], [32, 19, 2],[53, 60, 44], [32, 17, 17, 2],[16, 16, 31, 31]);txt = getActiveGroup(gcbh);text(2, 100, txt,'verticalAlignment', 'top');
  Signal Builder3 : Subsystem  Tag=STV Subsys  Commented=on  LoadFcn=sigbuilder_block('load');  StartFcn=sigbuilder_block('start');  StopFcn=sigbuilder_block('stop');  ClipboardFcn=sigbuilder_block('clipboard');  mask(Sigbuilder block){tuvar=[0:10]}
      mask help: Simulink:masks:SigbuilderBlock_MD
      mask init:
      | if ~strcmp(get_param(bdroot(gcbh),'SimulationStatus'),'stopped') tuvar = sigbuilder_block('maskInit'); end
      settings: CopyFcn=sigbuilder_block('copy');  DeleteFcn=sigbuilder_block('delete');  ModelCloseFcn=sigbuilder_block('modelClose');  PreSaveFcn=sigbuilder_block('preSave');  PauseFcn=sigbuilder_block('pause');  ContinueFcn=sigbuilder_block('continue');  NameChangeFcn=sigbuilder_block('namechange');  OpenFcn=sigbuilder_block('open',[437.6 199.2 550.4 400 ]);  CloseFcn=sigbuilder_block('close');
      mask Display: plot(0, 0, 100, 100,[2, 2, 32, 32, 2], [68, 8, 8, 68, 68],[32, 2], [38, 38], [32, 19, 2],[53, 60, 44], [32, 17, 17, 2],[16, 16, 31, 31]);txt = getActiveGroup(gcbh);text(2, 100, txt,'verticalAlignment', 'top');
  Signal Builder4 : Subsystem  Tag=STV Subsys  Commented=on  LoadFcn=sigbuilder_block('load');  StartFcn=sigbuilder_block('start');  StopFcn=sigbuilder_block('stop');  ClipboardFcn=sigbuilder_block('clipboard');  mask(Sigbuilder block){tuvar=[0:10]}
      mask help: Simulink:masks:SigbuilderBlock_MD
      mask init:
      | if ~strcmp(get_param(bdroot(gcbh),'SimulationStatus'),'stopped') tuvar = sigbuilder_block('maskInit'); end
      settings: CopyFcn=sigbuilder_block('copy');  DeleteFcn=sigbuilder_block('delete');  ModelCloseFcn=sigbuilder_block('modelClose');  PreSaveFcn=sigbuilder_block('preSave');  PauseFcn=sigbuilder_block('pause');  ContinueFcn=sigbuilder_block('continue');  NameChangeFcn=sigbuilder_block('namechange');  OpenFcn=sigbuilder_block('open',[437.6 199.2 550.4 400 ]);  CloseFcn=sigbuilder_block('close');
      mask Display: plot(0, 0, 100, 100,[2, 2, 32, 32, 2], [68, 8, 8, 68, 68],[32, 2], [38, 38], [32, 19, 2],[53, 60, 44], [32, 17, 17, 2],[16, 16, 31, 31]);txt = getActiveGroup(gcbh);text(2, 100, txt,'verticalAlignment', 'top');
  Sine Wave{1..2,5..6} (4 alike) : Sin  Amplitude=0.1  Bias=0.1  Frequency=2*pi  SampleTime=0.01
  Sine Wave{3..4,7..8} (4 alike) : Sin  Commented=on  Amplitude=0.1  Bias=0.1  Frequency=2*pi  SampleTime=0.01
  Step{1..4} (4 alike) : Step  After=0.1  SampleTime=0
  Subsystem1 : Subsystem  Commented=on  mask{e_kp=3, e_ki=0, e_kd=0}
  Subsystem2 : Subsystem  mask{e_kp=3, e_ki=0, e_kd=0}
  Subsystem3 : Subsystem  mask{e_kp=0, e_ki=0, e_kd=0}
  Subsystem4 : Subsystem  Commented=on  mask{e_kp=0, e_ki=0, e_kd=0}
  Sum1 : Sum  Inputs=+-+-
  Sum{8,10,13..14,24,29,36,41} (8 alike) : Sum  Inputs=+|+|+
  Sum{23,28,100,108} (4 alike) : Sum  Inputs=-+-
  Sum{2..4,9,12,20..21,27,31..32,39,43,98,101,103..104} (16 alike) : Sum  Inputs=|+-
  Sum{5,7,11,22,25..26,33..34,37..38,95,102,105..106} (14 alike) : Sum  Inputs=-+|
  Sum15 : Sum  Commented=on  Inputs=+-+-
  Sum{16,51..52,58,63,71,77,83} (8 alike) : Sum  Commented=on  Inputs=+|+|+
  Sum{17,48,57,62} (4 alike) : Sum  Commented=on  Inputs=-+-
  Sum{18,44..45,50,53..55,61,64,66..67,74..75,79,84,86} (16 alike) : Sum  Commented=on  Inputs=|+-
  Sum{19,46..47,49,56,59..60,68..69,72..73,80,82,85} (14 alike) : Sum  Commented=on  Inputs=-+|
  Sum30 : Sum  Inputs=++|
  Sum35 : Sum  Inputs=-+-+
  Sum40 : Sum  Inputs=+-+-
  Sum42 : Sum  Inputs=++|
  Sum6 : Sum  Inputs=-+-+
  Sum65 : Sum  Commented=on  Inputs=++|
  Sum70 : Sum  Commented=on  Inputs=-+-+
  Sum76 : Sum  Commented=on  Inputs=+-+-
  Sum78 : Sum  Commented=on  Inputs=++|
  Sum81 : Sum  Commented=on  Inputs=-+-+
  Transfer Fcn{,7,9..10} (4 alike) : TransferFcn  Numerator=[1 0 0]  Denominator=[tao^2 2*tao 1]
  Transfer Fcn{1..3,5..6,8,13..14} (8 alike) : TransferFcn  Denominator=[L R]
  Transfer Fcn{11,15..20,22} (8 alike) : TransferFcn  Commented=on  Denominator=[L R]
  Transfer Fcn{4,12,21,23} (4 alike) : TransferFcn  Commented=on  Numerator=[1 0 0]  Denominator=[tao^2 2*tao 1]
  adrc无前馈 : Gain
  adrc无前馈1 : Gain  Commented=on
  adrc有前馈 : Gain
  adrc有前馈1 : Gain  Commented=on
  pid无前馈 : Gain
  pid无前馈1 : Gain  Commented=on
  pid有前馈 : Gain
  pid有前馈1 : Gain  Commented=on
  二阶adrc1 : Subsystem  Commented=on  mask{bo=180, wo=500, wc=140}
      mask prompts: bo "补偿系数bo"; wo "观测器带宽wo"; wc "控制器带宽wc"
      mask init:
      | a_kp = wc^2;
      | a_kd = 2*wc;
      | beta1 = 3*wo;
      | beta2 = 3*wo^2;
      | beta3 = wo^3;
  二阶adrc2 : Subsystem  Commented=on  mask{bo=180, wo=500, wc=140}
      mask prompts: bo "补偿系数bo"; wo "观测器带宽wo"; wc "控制器带宽wc"
      mask init:
      | a_kp = wc^2;
      | a_kd = 2*wc;
      | beta1 = 3*wo;
      | beta2 = 3*wo^2;
      | beta3 = wo^3;
  二阶adrc3 : Subsystem  mask{bo=180, wo=400, wc=140}
      mask prompts: bo "补偿系数bo"; wo "观测器带宽wo"; wc "控制器带宽wc"
      mask init:
      | a_kp = wc^2;
      | a_kd = 2*wc;
      | beta1 = 3*wo;
      | beta2 = 3*wo^2;
      | beta3 = wo^3;
  二阶adrc4 : Subsystem  Commented=on  mask{bo=110, wo=500, wc=140}
      mask prompts: bo "补偿系数bo"; wo "观测器带宽wo"; wc "控制器带宽wc"
      mask init:
      | a_kp = wc^2;
      | a_kd = 2*wc;
      | beta1 = 3*wo;
      | beta2 = 3*wo^2;
      | beta3 = wo^3;
  二阶adrc5 : Subsystem  mask{bo=180, wo=400, wc=140}
      mask prompts: bo "补偿系数bo"; wo "观测器带宽wo"; wc "控制器带宽wc"
      mask init:
      | a_kp = wc^2;
      | a_kd = 2*wc;
      | beta1 = 3*wo;
      | beta2 = 3*wo^2;
      | beta3 = wo^3;
  二阶adrc6 : Subsystem  mask{bo=110, wo=500, wc=140}
      mask prompts: bo "补偿系数bo"; wo "观测器带宽wo"; wc "控制器带宽wc"
      mask init:
      | a_kp = wc^2;
      | a_kd = 2*wc;
      | beta1 = 3*wo;
      | beta2 = 3*wo^2;
      | beta3 = wo^3;
  二阶adrc7 : Subsystem  mask{bo=110, wo=500, wc=140}
      mask prompts: bo "补偿系数bo"; wo "观测器带宽wo"; wc "控制器带宽wc"
      mask init:
      | a_kp = wc^2;
      | a_kd = 2*wc;
      | beta1 = 3*wo;
      | beta2 = 3*wo^2;
      | beta3 = wo^3;
  二阶adrc8 : Subsystem  Commented=on  mask{bo=110, wo=500, wc=140}
      mask prompts: bo "补偿系数bo"; wo "观测器带宽wo"; wc "控制器带宽wc"
      mask init:
      | a_kp = wc^2;
      | a_kd = 2*wc;
      | beta1 = 3*wo;
      | beta2 = 3*wo^2;
      | beta3 = wo^3;
  前馈补偿 : MATLAB Function  TreatAsAtomicUnit=on
  前馈补偿1 : MATLAB Function  Commented=on  TreatAsAtomicUnit=on
  前馈补偿2 : MATLAB Function  TreatAsAtomicUnit=on
  前馈补偿3 : MATLAB Function  Commented=on  TreatAsAtomicUnit=on
  同 : Subsystem
  同1 : Subsystem
  同2 : Subsystem  Commented=on
  同3 : Subsystem
  同4 : Subsystem
  同5 : Subsystem  Commented=on
  同6 : Subsystem  Commented=on
  同7 : Subsystem  Commented=on
  滑动摩擦模型1 : MATLAB Function  TreatAsAtomicUnit=on
  滑动摩擦模型2 : MATLAB Function  TreatAsAtomicUnit=on
  滑动摩擦模型3 : MATLAB Function  TreatAsAtomicUnit=on
  滑动摩擦模型4 : MATLAB Function  TreatAsAtomicUnit=on
  滑动摩擦模型5 : MATLAB Function  Commented=on  TreatAsAtomicUnit=on
  滑动摩擦模型6 : MATLAB Function  Commented=on  TreatAsAtomicUnit=on
  滑动摩擦模型7 : MATLAB Function  Commented=on  TreatAsAtomicUnit=on
  滑动摩擦模型8 : MATLAB Function  Commented=on  TreatAsAtomicUnit=on
  相反 : Subsystem
  相反1 : Subsystem
  相反2 : Subsystem  Commented=on
  相反3 : Subsystem
  相反4 : Subsystem
  相反5 : Subsystem  Commented=on
  相反6 : Subsystem  Commented=on
  相反7 : Subsystem  Commented=on
  龙门平台1 : MATLAB Function  TreatAsAtomicUnit=on
  龙门平台2 : MATLAB Function  TreatAsAtomicUnit=on
  龙门平台3 : MATLAB Function  TreatAsAtomicUnit=on
  龙门平台4 : MATLAB Function  TreatAsAtomicUnit=on
  龙门平台5 : MATLAB Function  Commented=on  TreatAsAtomicUnit=on
  龙门平台6 : MATLAB Function  Commented=on  TreatAsAtomicUnit=on
  龙门平台7 : MATLAB Function  Commented=on  TreatAsAtomicUnit=on
  龙门平台8 : MATLAB Function  Commented=on  TreatAsAtomicUnit=on
  wires:
  Gain24/1 -> Sum22/1
  Integrator9/1 -> Gain22/1, Sum27/2, Gain20/1, Integrator10/1  "速度反馈"
  Gain23/1 -> Sum29/2
  Integrator12/1 -> Add3/1, Subsystem2/1(位置反馈1), 二阶adrc3/2(y)  "位置反馈1"
  Transfer Fcn6/1 -> Sum25/1, Gain23/1  "电流反馈"
  Sum23/1 -> 龙门平台3/1(u1)
  Gain20/1 -> Sum28/3
  Band-Limited White Noise6/1 -> Gain21/1
  二阶adrc3/1(u) -> Sum26/2
  PID Controller7/1 -> Sum22/2
  PID Controller4/1 -> Sum31/1
  PID Controller8/1 -> Sum20/1
  Integrator10/1 -> Add3/2, Subsystem2/2(位置反馈2), 二阶adrc5/2(y)  "位置反馈1"
  Sum31/1 -> Transfer Fcn6/1
  Gain21/1 -> Sum24/1
  Sum28/1 -> 龙门平台3/3(u2)
  相反3/1(Out1) -> Sum29/1
  同3/1(Out1) -> Sum24/3
  Integrator11/1 -> Sum26/1, Gain24/1, Gain19/1, Integrator12/1
  滑动摩擦模型3/1(f1) -> Sum23/3
  Sum27/1 -> PID Controller6/1
  Gain19/1 -> Sum23/1
  Sum22/1 -> Transfer Fcn5/1
  Subsystem2/1(error) -> Sum30/1, Sum21/2
  Step3/1 -> Sum30/2, Sum21/1  "输入"
  Band-Limited White Noise5/1 -> Gain18/1
  Gain18/1 -> Sum29/3
  Sum30/1 -> 二阶adrc5/1(p)
  Gain17/1 -> Sum24/2
  Sum26/1 -> PID Controller8/1
  Sum25/1 -> PID Controller4/1
  Transfer Fcn5/1 -> Sum20/2, Gain17/1  "电流反馈"
  Gain22/1 -> Sum31/2
  龙门平台3/2(out2) -> Integrator9/1
  二阶adrc5/1(u) -> Sum27/1
  Sum20/1 -> PID Controller7/1
  Add3/1 -> adrc无前馈/1  "同步误差"
  滑动摩擦模型3/2(f2) -> Sum28/1
  龙门平台3/1(out1) -> Integrator11/1
  Sine Wave5/1 -> 滑动摩擦模型3/1(y), 龙门平台3/2(y)
  Sum29/1 -> Sum28/2
  Sum21/1 -> 二阶adrc3/1(p)
  Sum24/1 -> Sum23/2
  PID Controller6/1 -> Sum25/2
  adrc无前馈/1 -> Scope/2
  PID Controller42/1 -> Sum105/2
  Transfer Fcn/1 -> Product/1
  Product1/1 -> Sum1/1
  Sine Wave1/1 -> 前馈补偿/1(y), 滑动摩擦模型1/1(y), 龙门平台1/2(y)
  PID Controller39/1 -> Sum103/1
  Integrator23/1 -> Add17/1, Sum95/1  "位置反馈1"
  Gain92/1 -> Sum8/2
  Product/1 -> Sum35/4
  Sum10/1 -> Sum1/3
  Integrator20/1 -> Integrator21/1, Sum103/2, Gain100/1, Gain95/1  "速度反馈"
  Sum32/1 -> PID Controller9/1
  前馈补偿/1(meq1) -> Product/2
  同/1(Out1) -> Sum8/3
  Gain4/1 -> 龙门平台1/3(u2)
  Transfer Fcn13/1 -> Sum104/2, Gain92/1  "电流反馈"
  PID Controller38/1 -> Sum102/2
  Sum105/1 -> PID Controller21/1
  龙门平台4/2(out2) -> Integrator20/1
  PID Controller21/1 -> Sum98/1
  Transfer Fcn2/1 -> Gain10/1, Sum33/1  "电流反馈"
  Gain/1 -> 龙门平台1/1(u1)
  Sum103/1 -> PID Controller42/1
  Sum11/1 -> PID Controller11/1
  Sum100/1 -> 龙门平台4/3(u2)
  PID Controller41/1 -> Sum104/1
  PID Controller13/1 -> Sum32/1
  Step1/1 -> Scope2/1, Sum11/2, Transfer Fcn/1, Sum2/1, Transfer Fcn7/1  "输入"
  Gain25/1 -> Sum36/1
  Sum108/1 -> 龙门平台4/1(u1)
  Sum101/1 -> PID Controller39/1
  Sum35/1 -> Gain/1
  Sum1/1 -> Gain4/1
  Integrator1/1 -> Sum9/2, Gain1/1, Gain8/1, Integrator2/1  "速度反馈"
  Transfer Fcn1/1 -> Gain5/1, Sum32/2  "电流反馈"
  Add17/1 -> pid无前馈/1  "同步误差"
  Transfer Fcn7/1 -> Product1/2
  Sum8/1 -> Sum108/2
  Gain94/1 -> Sum108/1
  Integrator22/1 -> Integrator23/1, Gain99/1, Sum102/1, Gain94/1
  Sum12/1 -> Transfer Fcn2/1
  PID Controller12/1 -> Sum9/1
  前馈补偿/2(meq2) -> Product1/1
  Gain95/1 -> Sum100/3
  PID Controller10/1 -> Sum12/1
  Sum7/1 -> PID Controller13/1
  PID Controller20/1 -> Sum106/2
  Sum98/1 -> Transfer Fcn14/1
  Sum102/1 -> PID Controller41/1
  Gain11/1 -> Sum34/1
  Sum95/1 -> PID Controller38/1
  Gain100/1 -> Sum98/2
  Gain1/1 -> Sum12/2
  Sum106/1 -> Transfer Fcn13/1
  Transfer Fcn14/1 -> Gain98/1, Sum105/1  "电流反馈"
  滑动摩擦模型1/1(f1) -> Sum35/3
  Gain5/1 -> Sum36/2
  Sum2/1 -> PID Controller12/1
  Gain98/1 -> Sum41/2
  PID Controller14/1 -> Sum33/2
  Sum9/1 -> PID Controller14/1
  Add1/1 -> pid有前馈/1  "同步误差"
  Sum34/1 -> Transfer Fcn1/1
  Band-Limited White Noise2/1 -> Gain25/1
  Sum36/1 -> Sum35/2
  龙门平台4/1(out1) -> Integrator22/1
  相反1/1(Out1) -> Sum10/1
  Integrator3/1 -> Gain11/1, Sum7/1, Gain7/1, Integrator4/1
  Integrator21/1 -> Sum101/2, Add17/2  "位置反馈1"
  Gain99/1 -> Sum106/1
  同1/1(Out1) -> Sum36/3
  龙门平台1/1(out1) -> Integrator3/1
  Sum33/1 -> PID Controller10/1
  Sum104/1 -> PID Controller20/1
  Gain6/1 -> Sum10/3
  Integrator4/1 -> Add1/1, Sum11/1  "位置反馈1"
  Sum41/1 -> Sum100/2
  Gain7/1 -> Sum35/1
  PID Controller11/1 -> Sum7/2
  滑动摩擦模型1/2(f2) -> Sum1/2
  相反/1(Out1) -> Sum41/1
  龙门平台1/2(out2) -> Integrator1/1
  Gain10/1 -> Sum10/2
  Integrator2/1 -> Sum2/2, Add1/2  "位置反馈1"
  Gain8/1 -> Sum1/4
  PID Controller9/1 -> Sum34/2
  Band-Limited White Noise1/1 -> Gain6/1
  pid有前馈/1 -> Scope/3
  pid无前馈/1 -> Scope/4
  Saturation1/1 -> Product3/2
  二阶adrc7/1(u) -> Sum39/1
  Transfer Fcn9/1 -> Saturation/1
  Transfer Fcn3/1 -> Sum3/2, Gain2/1  "电流反馈"
  PID Controller1/1 -> Sum37/2
  Sum3/1 -> PID Controller2/1
  Gain28/1 -> Sum40/4
  Transfer Fcn10/1 -> Saturation1/1
  滑动摩擦模型2/2(f2) -> Sum40/2
  Product2/1 -> Sum6/4
  Sum42/1 -> 二阶adrc7/1(p)
  前馈补偿2/2(meq2) -> Product3/1
  Saturation/1 -> Product2/1
  相反4/1(Out1) -> Sum14/1
  Sum38/1 -> PID Controller3/1
  Gain26/1 -> Sum14/3
  Band-Limited White Noise7/1 -> Gain26/1
  Gain2/1 -> Sum13/2
  Gain32/1 -> Sum5/1
  Gain31/1 -> Sum14/2
  Product3/1 -> Sum40/1
  Integrator13/1 -> Gain30/1, Sum39/2, Gain28/1, Integrator14/1  "速度反馈"
  Sum14/1 -> Sum40/3
  Step4/1 -> Sum42/2, Sum4/1  "输入"
  Integrator16/1 -> Transfer Fcn9/1, Subsystem3/1(位置反馈1), 二阶adrc6/2(y), Scope6/1, Add4/1  "位置反馈1"
  Integrator15/1 -> Sum38/1, Gain32/1, Gain27/1, Integrator16/1
  Add4/1 -> adrc有前馈/1  "同步误差"
  龙门平台2/2(out2) -> Integrator13/1
  Gain27/1 -> Sum6/1
  Subsystem3/1(error) -> Sum42/1, Sum4/2
  Band-Limited White Noise8/1 -> Gain29/1
  前馈补偿2/1(meq1) -> Product2/2
  龙门平台2/1(out1) -> Integrator15/1
  Sum6/1 -> 龙门平台2/1(u1)
  Gain30/1 -> Sum43/2
  Sum40/1 -> 龙门平台2/3(u2)
  Sum4/1 -> 二阶adrc6/1(p)
  Sum37/1 -> PID Controller5/1
  Sum5/1 -> Transfer Fcn3/1
  Sine Wave6/1 -> Scope5/1, 滑动摩擦模型2/1(y), 前馈补偿2/1(y), 龙门平台2/2(y)
  同4/1(Out1) -> Sum13/3
  Sum39/1 -> PID Controller1/1
  滑动摩擦模型2/1(f1) -> Sum6/3
  Sum13/1 -> Sum6/2
  PID Controller2/1 -> Sum5/2
  PID Controller3/1 -> Sum3/1
  Gain29/1 -> Sum13/1
  Integrator14/1 -> Transfer Fcn10/1, 二阶adrc7/2(y), Subsystem3/2(位置反馈2), Add4/2  "位置反馈1"
  Sum43/1 -> Transfer Fcn8/1
  adrc有前馈/1 -> Scope/1
  Transfer Fcn8/1 -> Sum37/1, Gain31/1  "电流反馈"
  PID Controller5/1 -> Sum43/1
  二阶adrc6/1(u) -> Sum38/2
  Band-Limited White Noise3/1 -> Gain3/1
  Gain3/1 -> Sum41/3
  Band-Limited White Noise4/1 -> Gain9/1
  Gain9/1 -> Sum8/1
  滑动摩擦模型4/1(f1) -> Sum108/3
  滑动摩擦模型4/2(f2) -> Sum100/1
  Sine Wave2/1 -> 滑动摩擦模型4/1(y), 龙门平台4/2(y)
  Step2/1 -> Sum101/1, Sum95/2
  Product6/1 -> Sum81/4
  Product4/1 -> Sum70/4
  滑动摩擦模型6/1(f1) -> Sum81/3
  Gain36/1 -> Sum51/2
  PID Controller18/1 -> Sum84/1
  Gain49/1 -> Sum52/2
  PID Controller15/1 -> Sum72/2
  Product7/1 -> Sum76/1
  Gain47/1 -> Sum77/3
  Gain50/1 -> Sum80/1
  Band-Limited White Noise12/1 -> Gain56/1
  Sum75/1 -> 二阶adrc4/1(p)
  Signal Builder3/1(Signal 1) -> Sum18/1, Sum85/2
  Transfer Fcn12/1 -> Saturation3/1
  Gain56/1 -> Sum83/1
  Sum84/1 -> PID Controller22/1
  Integrator26/1 -> Integrator27/1, Sum44/2, Gain15/1, Gain59/1  "速度反馈"
  Sum57/1 -> 龙门平台7/1(u1)
  Integrator18/1 -> Add7/2, Transfer Fcn12/1, 二阶adrc8/2(y), Subsystem4/2(位置反馈2)  "位置反馈1"
  Band-Limited White Noise11/1 -> Gain47/1
  滑动摩擦模型5/2(f2) -> Sum15/2
  Signal Builder1/1(Signal 1) -> Sum65/2, Sum55/1  "输入"
  Sum15/1 -> Gain51/1
  Sum72/1 -> PID Controller32/1
  Transfer Fcn22/1 -> Sum72/1, Gain49/1  "电流反馈"
  PID Controller23/1 -> Sum80/2
  Sum79/1 -> Transfer Fcn22/1
  Gain51/1 -> 龙门平台5/3(u2)
  Gain34/1 -> Sum63/3
  Sum47/1 -> Transfer Fcn15/1
  Gain45/1 -> Sum76/4
  Sum81/1 -> 龙门平台6/1(u1)
  Gain46/1 -> Sum51/1
  龙门平台7/2(out2) -> Integrator32/1
  Saturation3/1 -> Product7/2
  Sum78/1 -> 二阶adrc8/1(p)
  Signal Builder4/1(Signal 1) -> Sum78/2, Sum75/1  "输入"
  Band-Limited White Noise16/1 -> Gain46/1
  Sum53/1 -> PID Controller18/1
  同7/1(Out1) -> Sum51/3
  PID Controller32/1 -> Sum79/1
  前馈补偿3/2(meq2) -> Product7/1
  Sum46/1 -> PID Controller25/1
  Gain48/1 -> Sum79/2
  相反7/1(Out1) -> Sum52/1
  龙门平台6/1(out1) -> Integrator19/1
  Sum51/1 -> Sum81/2
  Integrator19/1 -> Sum73/1, Gain50/1, Gain44/1, Integrator24/1
  Integrator24/1 -> Add7/1, Transfer Fcn23/1, Subsystem4/1(位置反馈1), 二阶adrc4/2(y)  "位置反馈1"
  前馈补偿1/2(meq2) -> Product5/1
  Gain43/1 -> Sum52/3
  前馈补偿3/1(meq1) -> Product6/2
  滑动摩擦模型8/1(f1) -> Sum48/3
  Gain39/1 -> Sum66/2
  相反2/1(Out1) -> Sum77/1
  Integrator17/1 -> Gain48/1, Sum74/2, Gain45/1, Integrator18/1  "速度反馈"
  龙门平台8/2(out2) -> Integrator26/1
  Integrator5/1 -> Sum84/2, Gain13/1, Gain55/1, Integrator25/1  "速度反馈"
  龙门平台6/2(out2) -> Integrator17/1
  滑动摩擦模型8/2(f2) -> Sum17/1
  Sum71/1 -> Sum70/2
  Sum74/1 -> PID Controller15/1
  Sine Wave8/1 -> 滑动摩擦模型6/1(y), 前馈补偿3/1(y), 龙门平台6/2(y)
  Sum73/1 -> PID Controller26/1
  Transfer Fcn21/1 -> Product5/2
  Transfer Fcn11/1 -> Gain52/1, Sum67/2  "电流反馈"
  Sum69/1 -> Transfer Fcn11/1
  PID Controller26/1 -> Sum64/1
  Integrator25/1 -> Sum53/2, Add2/2  "位置反馈1"
  Sum48/1 -> 龙门平台8/1(u1)
  滑动摩擦模型6/2(f2) -> Sum76/2
  Saturation2/1 -> Product6/1
  Integrator28/1 -> Integrator29/1, Gain61/1, Sum19/1, Gain58/1
  PID Controller22/1 -> Sum68/2
  Transfer Fcn18/1 -> Sum64/2, Gain36/1  "电流反馈"
  Sum52/1 -> Sum76/3
  pid无前馈1/1 -> Scope1/4
  Gain14/1 -> Sum16/2
  Gain54/1 -> Sum70/1
  Gain44/1 -> Sum81/1
  Sum45/1 -> PID Controller24/1
  Sum77/1 -> Sum17/2
  Gain58/1 -> Sum48/1
  Integrator32/1 -> Sum61/2, Gain39/1, Gain37/1, Integrator6/1  "速度反馈"
  Gain57/1 -> Sum83/2
  同5/1(Out1) -> Sum71/3
  Integrator8/1 -> Add6/1, Subsystem1/1(位置反馈1), 二阶adrc1/2(y)  "位置反馈1"
  Gain53/1 -> Sum16/3
  Integrator27/1 -> Sum18/2, Add5/2  "位置反馈1"
  Gain52/1 -> Sum71/2
  Sum80/1 -> Transfer Fcn18/1
  龙门平台8/1(out1) -> Integrator28/1
  Gain13/1 -> Sum50/2
  龙门平台5/1(out1) -> Integrator30/1
  Integrator30/1 -> Gain16/1, Sum82/1, Gain54/1, Integrator31/1
  Band-Limited White Noise15/1 -> Gain43/1
  相反5/1(Out1) -> Sum16/1
  Transfer Fcn16/1 -> Gain60/1, Sum46/1  "电流反馈"
  Band-Limited White Noise13/1 -> Gain34/1
  Add2/1 -> pid有前馈1/1  "同步误差"
  二阶adrc4/1(u) -> Sum73/2
  Gain61/1 -> Sum47/1
  Gain55/1 -> Sum15/4
  Sum76/1 -> Scope4/1, 龙门平台6/3(u2)
  Sum85/1 -> PID Controller27/1
  pid有前馈1/1 -> Scope1/3
  Gain59/1 -> Sum17/3
  Sum83/1 -> Sum48/2
  二阶adrc1/1(u) -> Sum60/2
  Sum18/1 -> PID Controller28/1
  adrc无前馈1/1 -> Scope1/2
  Gain16/1 -> Sum69/1
  Sum50/1 -> Transfer Fcn17/1
  PID Controller24/1 -> Sum47/2
  Add5/1 -> pid无前馈1/1  "同步误差"
  Signal Builder2/1(Signal 1) -> Scope3/1, Sum49/2, Transfer Fcn4/1, Sum53/1, Transfer Fcn21/1  "输入"
  Gain15/1 -> Sum86/2
  Subsystem4/1(error) -> Sum78/1, Sum75/2
  Sum86/1 -> Transfer Fcn16/1
  PID Controller28/1 -> Sum44/1
  PID Controller19/1 -> Sum67/1
  Transfer Fcn23/1 -> Saturation2/1
  Gain42/1 -> Sum71/1
  Add6/1 -> adrc无前馈1/1  "同步误差"
  Sum49/1 -> PID Controller17/1
  Gain60/1 -> Sum77/2
  Sum67/1 -> PID Controller36/1
  Band-Limited White Noise10/1 -> Gain42/1
  Sum44/1 -> PID Controller31/1
  PID Controller17/1 -> Sum82/2
  PID Controller27/1 -> Sum19/2
  PID Controller36/1 -> Sum69/2
  前馈补偿1/1(meq1) -> Product4/2
  Sum64/1 -> PID Controller23/1
  PID Controller25/1 -> Sum86/1
  Transfer Fcn15/1 -> Sum45/2, Gain57/1  "电流反馈"
  Gain12/1 -> 龙门平台5/1(u1)
  Sum68/1 -> PID Controller16/1
  Sum55/1 -> 二阶adrc1/1(p)
  Sine Wave3/1 -> 前馈补偿1/1(y), 滑动摩擦模型5/1(y), 龙门平台5/2(y)
  Subsystem1/1(error) -> Sum65/1, Sum55/2
  Transfer Fcn17/1 -> Gain14/1, Sum68/1  "电流反馈"
  PID Controller16/1 -> Sum50/1
  Transfer Fcn19/1 -> Sum54/2, Gain33/1  "电流反馈"
  Product5/1 -> Sum15/1
  Sum58/1 -> Sum57/2
  Sum63/1 -> Sum62/2
  Sum70/1 -> Gain12/1
  Integrator31/1 -> Add2/1, Sum49/1  "位置反馈1"
  滑动摩擦模型7/2(f2) -> Sum62/1
  Integrator7/1 -> Sum60/1, Gain41/1, Gain35/1, Integrator8/1
  龙门平台5/2(out2) -> Integrator5/1
  Gain38/1 -> Sum58/1
  Sum61/1 -> PID Controller33/1
  Sum62/1 -> 龙门平台7/3(u2)
  Sum54/1 -> PID Controller34/1
  Sum60/1 -> PID Controller35/1
  Gain33/1 -> Sum58/2
  二阶adrc2/1(u) -> Sum61/1
  Transfer Fcn20/1 -> Sum59/1, Gain40/1  "电流反馈"
  Sine Wave7/1 -> 滑动摩擦模型7/1(y), 龙门平台7/2(y)
  PID Controller33/1 -> Sum59/2
  Integrator29/1 -> Add5/1, Sum85/1  "位置反馈1"
  adrc有前馈1/1 -> Scope1/1
  Add7/1 -> adrc有前馈1/1  "同步误差"
  Gain35/1 -> Sum57/1
  Sum65/1 -> 二阶adrc2/1(p)
  滑动摩擦模型7/1(f1) -> Sum57/3
  二阶adrc8/1(u) -> Sum74/1
  相反6/1(Out1) -> Sum63/1
  PID Controller35/1 -> Sum54/1
  Band-Limited White Noise14/1 -> Gain38/1
  Band-Limited White Noise9/1 -> Gain53/1
  PID Controller29/1 -> Sum66/1
  Sum17/1 -> 龙门平台8/3(u2)
  Sum82/1 -> PID Controller19/1
  Transfer Fcn4/1 -> Product4/1
  PID Controller31/1 -> Sum46/2
  Gain37/1 -> Sum62/3
  龙门平台7/1(out1) -> Integrator7/1
  Sum16/1 -> Sum15/3
  Gain40/1 -> Sum63/2
  Integrator6/1 -> Add6/2, Subsystem1/2(位置反馈2), 二阶adrc2/2(y)  "位置反馈1"
  PID Controller30/1 -> Sum45/1
  Sum56/1 -> Transfer Fcn19/1
  滑动摩擦模型5/1(f1) -> Sum70/3
  同2/1(Out1) -> Sum83/3
  Sum66/1 -> Transfer Fcn20/1
  PID Controller34/1 -> Sum56/2
  Sine Wave4/1 -> 滑动摩擦模型8/1(y), 龙门平台8/2(y)
  Gain41/1 -> Sum56/1
  Sum19/1 -> PID Controller30/1
  同6/1(Out1) -> Sum58/3
  Sum59/1 -> PID Controller29/1
